simulink model "SDOFmodel"  (R2018a)
settings: Solver=VariableStepAuto  StartTime=0.0  StopTime=2.56  RelTol=1e-3
values from neighbouring files (symbols this model uses):
  c = 2000    [suspensiondata.mat]
  M = 1000    [fullcar_values.m]    (also in suspensiondata.mat)
settings Model: Creator=Dev  LastModifiedBy=Saurabh Suman

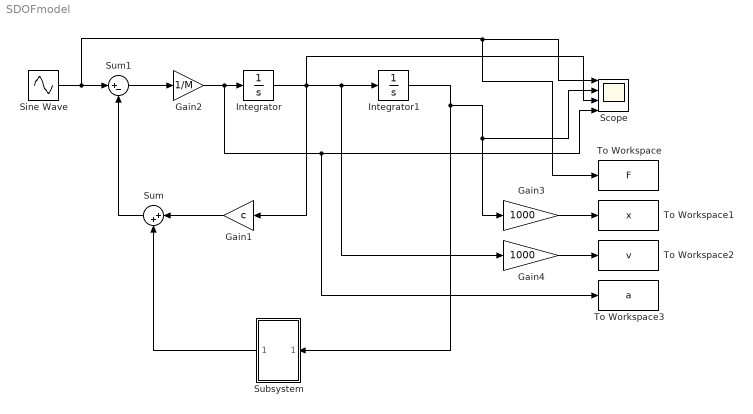
== system SDOFmodel ==
  Gain1 : Gain  Gain=c
  Gain2 : Gain  Gain=1/M
  Gain3 : Gain  Gain=1000
  Gain4 : Gain  Gain=1000
  Integrator : Integrator
  Integrator1 : Integrator
  Scope : Scope  NumInputPorts=4
  Sine Wave : Sin  Frequency=31.4  SampleTime=0.001
  Subsystem : Subsystem
  Sum : Sum  Inputs=|++
  Sum1 : Sum  Inputs=|+-
  To Workspace : ToWorkspace  VariableName=F  SaveFormat=Timeseries  SampleTime=-1
  To Workspace1 : ToWorkspace  VariableName=x  SaveFormat=Timeseries  SampleTime=-1
  To Workspace2 : ToWorkspace  VariableName=v  SaveFormat=Timeseries  SampleTime=-1
  To Workspace3 : ToWorkspace  VariableName=a  SaveFormat=Timeseries  SampleTime=-1
  wires:
  Integrator/1 -> Scope/3, Gain1/1, Gain4/1, Integrator1/1
  Integrator1/1 -> Subsystem/1(In3), Gain3/1, Scope/2
  Sine Wave/1 -> To Workspace/1, Scope/1, Sum1/1
  Sum/1 -> Sum1/2
  Sum1/1 -> Gain2/1
  Gain2/1 -> To Workspace3/1, Scope/4, Integrator/1
  Gain3/1 -> To Workspace1/1
  Gain4/1 -> To Workspace2/1
  Gain1/1 -> Sum/1
  Subsystem/1(Out1) -> Sum/2

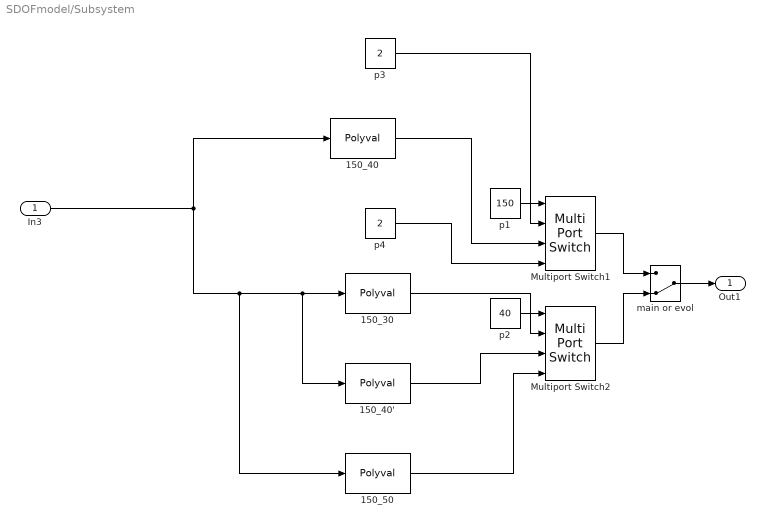
== system SDOFmodel/Subsystem ==
  In3 : Inport
  150_30 : Polyval  Coefs=[ -5.674e+09*6, 1.562e+09*5, -1.485e+08*4, 6.452e+06*3, -1.365e+05*2, 3607 ]
  150_40 : Polyval  Coefs=[ -4.597e+09*6, 1.259e+09*5, -1.21e+08*4, 5.755e+06*3, -1.495e+05*2, 4352 ]
  150_40' : Polyval  Coefs=[ -4.597e+09*6, 1.259e+09*5, -1.21e+08*4, 5.755e+06*3, -1.495e+05*2, 4352 ]
  150_50 : Polyval  Coefs=[ -1.771e+09*6, 3.133e+08*5, -5.807e+06*4, -4.747e+05*3, 187.7*2, 3121 ]
  Multiport Switch1 : MultiPortSwitch  DataPortOrder=Specify indices  DataPortIndices={200,150,100}
  Multiport Switch2 : MultiPortSwitch  DataPortOrder=Specify indices  DataPortIndices={30,40,50}
  main or evol : ManualSwitch  CurrentSetting=0
  p1 : Constant  Value=150
  p2 : Constant  Value=40
  p3 : Constant  Value=2
  p4 : Constant  Value=2
  Out1 : Outport
  wires:
  In3/1 -> 150_50/1, 150_40'/1, 150_30/1, 150_40/1
  p3/1 -> Multiport Switch1/2
  Multiport Switch1/1 -> main or evol/1
  Multiport Switch2/1 -> main or evol/2
  main or evol/1 -> Out1/1
  150_30/1 -> Multiport Switch2/2
  p1/1 -> Multiport Switch1/1
  p4/1 -> Multiport Switch1/4
  p2/1 -> Multiport Switch2/1
  150_40'/1 -> Multiport Switch2/3
  150_50/1 -> Multiport Switch2/4
  150_40/1 -> Multiport Switch1/3
